simulink model "rpi_driver_blocks"  (R2018b)
settings: Solver=ode45  StartTime=0.0  StopTime=10.0  RelTol=1e-3
PreLoadFcn:
  | Ts = 1e-3
PreSaveFcn:
  | set_param(gcs, 'location', [15 50 815 560])
settings Model: SimulationMode=external  ExtModeTrigDuration=100  Creator=The MathWorks Inc.  LastModifiedBy=benkl
settings DataIOCC: LimitDataPoints=on  SaveFormat=Array
settings OptimizationCC: BlockReduction=off  BooleanDataType=off  LifeSpan=inf
settings DebuggingCC: SaveWithParameterizedLinksMsg=none  UnderspecifiedInitializationDetection=Classic  MergeDetectMultiDrivingBlocksExec=none  SignalResolutionControl=TryResolveAllWithWarning  SFUnexpectedBacktrackingDiag=warning  SFNoUnconditionalDefaultTransitionDiag=warning  SFExecutionAtInitializationDiag=none
settings HardwareCC: ProdBitPerPointer=32  ProdBitPerSizeT=32  ProdBitPerPtrDiffT=32  ProdLargestAtomicFloat=None  ProdIntDivRoundTo=Undefined  ProdEndianess=Unspecified  ProdWordSize=32  ProdHWDeviceType=32-bit Generic  TargetUnknown=on
settings ModelReferenceCC: PropagateSignalLabelsOutOfModel=off
settings SFSimCC: SimUseLocalCustomCode=off
settings RTWCC: RTWUseLocalCustomCode=off
settings CodeAppCC: StateflowObjectComments=on
settings GRTTargetCC: TargetLangStandard=C89/C90 (ANSI)  GeneratePreprocessorConditionals=Disable all
settings ConfigComp: CovMetricSettings=dw  CovHtmlReporting=on  CovSaveCumulativeToWorkspaceVar=on  CovSaveSingleToWorkspaceVar=on  CovExternalEMLEnable=off  CovSFcnEnable=off

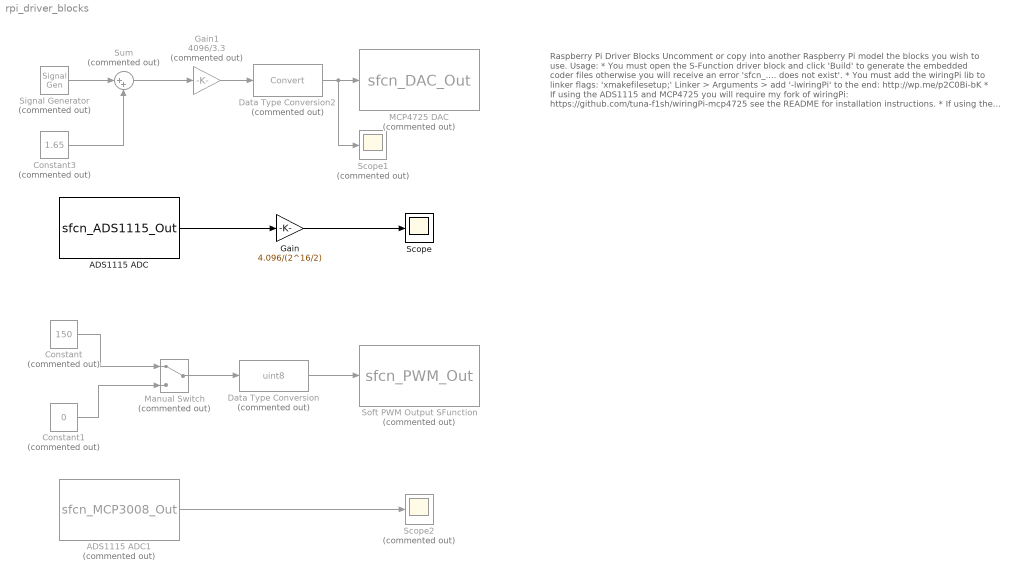
== system rpi_driver_blocks ==
  note: Raspberry Pi Driver Blocks
      |
      | Uncomment or copy into another Raspberry Pi model the blocks you wish to use.
      |
      | Usage:
      |
      | * You must open the S-Function driver block and click 'Build' to generate the embedded coder files
      | otherwise you will receive an error 'sfcn_.... does not exist'.
      |
      | * You must add the wiringPi lib to linker flags: 'xmakefilesetup;' Linker > Arguments > add '-lwiringPi' to the end:
      | http://wp.me/p2C0Bi-bK
      |
      | * If using the ADS1115 and MCP4725 you will require my fork of wiringPi: https://github.com/tuna-f1sh/wiringPi-mcp4725
      | see the README for installation instructions.
      |
      | * If using the PWM block, you will need to enable SPI in Raspbian - see:
      | http://uk.mathworks.com/help/supportpkg/raspberrypiio/examples/analog-input-using-spi.html or enable via SSH
      |
      | * The scopes work in real-time on the Pi to see the correct data is going to/coming from blocks.
      |
      | * The discrete timestep is set to 'Ts' throughout the model. This is initialised as 1e-3s at model load - it seems to be the
      | sweet spot for performance/usage. Remember to consider quantisation that this can create with signals driving the blocks.
      |
      | Notes:
      |
      | * wiringPi softPWM: https://projects.drogon.net/raspberry-pi/wiringpi/software-pwm-library/
      |
      | * Do not sure both ADC blocks at once without changing the wiringPi 'pin' assignment - it won't work.
      |
      | www.jbrengineering.co.uk - @j_whittington - 2015
  ADS1115 ADC : S-Function  InitFcn=try, set_param(gcb,'FunctionName','sfcn_ADS1115_Out'), end  FunctionName=sfcn_ADS1115_Out  Parameters=uint8(0)  SFunctionModules=sfcn_ADS1115_Out_wrapper  SFunctionDeploymentMode=off  EnableBusSupport=off  mask(S-Function Builder){}
      mask init:
      | val = [[.9  0.75 0.75 1 1 .9 .9 1]',[1 1 0.75 0.75 .9 .9 1 .9]'];try , sys = get_param(gcb,'SfunBuilderFcnName');if isempty(sys), sys = get_param(gcb,'FunctionName'); end,catch, sys = get_param(gcb,'FunctionName'); end
      settings: CopyFcn=set_param(gcbh,'LinkStatus','none')  PreSaveFcn=try, set_param(gcb,'FunctionName','sfcn_ADS1115_Out'), end  OpenFcn=sfunctionwizard(gcbh)
      mask Display: plot(val(:,1),val(:,2)),disp(sys), port_label('output',1,'y0')
  ADS1115 ADC1 : S-Function  Commented=on  InitFcn=try, set_param(gcb,'FunctionName','sfcn_MCP3008_Out'), end  FunctionName=sfcn_MCP3008_Out  Parameters=uint8(0)  SFunctionModules=sfcn_MCP3008_Out_wrapper  SFunctionDeploymentMode=off  EnableBusSupport=off  mask(S-Function Builder){}
      mask init: same as rpi_driver_blocks/ADS1115 ADC
      settings: CopyFcn=set_param(gcbh,'LinkStatus','none')  PreSaveFcn=try, set_param(gcb,'FunctionName','sfcn_MCP3008_Out'), end  OpenFcn=sfunctionwizard(gcbh)
      mask Display: plot(val(:,1),val(:,2)),disp(sys), port_label('output',1,'y0')
  Constant : Constant  Commented=on  Value=150
  Constant1 : Constant  Commented=on  Value=0
  Constant3 : Constant  Commented=on  Value=1.65  SampleTime=Ts
  Data Type Conversion : DataTypeConversion  Commented=on  OutDataTypeStr=uint8
  Data Type Conversion2 : DataTypeConversion  Commented=on
  Gain : Gain  Gain=4.096/(2^16/2)  SampleTime=Ts
  Gain1 : Gain  Commented=on  Gain=4096/3.3  SampleTime=Ts
  MCP4725 DAC : S-Function  Commented=on  InitFcn=try, set_param(gcb,'FunctionName','sfcn_DAC_Out'), end  FunctionName=sfcn_DAC_Out  Parameters=uint8(0)  SFunctionModules=sfcn_DAC_Out_wrapper  SFunctionDeploymentMode=off  EnableBusSupport=off  mask(S-Function Builder){}
      mask init: same as rpi_driver_blocks/ADS1115 ADC
      settings: CopyFcn=set_param(gcbh,'LinkStatus','none')  PreSaveFcn=try, set_param(gcb,'FunctionName','sfcn_DAC_Out'), end  OpenFcn=sfunctionwizard(gcbh)
      mask Display: plot(val(:,1),val(:,2)),disp(sys), port_label('input',1,'u0')
  Manual Switch : ManualSwitch  Commented=on
  Scope : Scope
  Scope1 : Scope  Commented=on
  Scope2 : Scope  Commented=on
  Signal Generator : SignalGenerator  Commented=on  Amplitude=1.65  Frequency=5
  Soft PWM Output SFunction : S-Function  Commented=on  InitFcn=try, set_param(gcb,'FunctionName','sfcn_PWM_Out'), end  FunctionName=sfcn_PWM_Out  Parameters=uint8(0)  SFunctionModules=sfcn_PWM_Out_wrapper  SFunctionDeploymentMode=off  EnableBusSupport=off  mask(S-Function Builder){}
      mask init: same as rpi_driver_blocks/ADS1115 ADC
      settings: CopyFcn=set_param(gcbh,'LinkStatus','none')  PreSaveFcn=try, set_param(gcb,'FunctionName','sfcn_PWM_Out'), end  OpenFcn=sfunctionwizard(gcbh)
      mask Display: plot(val(:,1),val(:,2)),disp(sys), port_label('input',1,'in')
  Sum : Sum  Commented=on  Inputs=|++
  wires:
  Constant/1 -> Manual Switch/1
  Constant1/1 -> Manual Switch/2
  Manual Switch/1 -> Data Type Conversion/1
  Data Type Conversion/1 -> Soft PWM Output SFunction/1
  Gain/1 -> Scope/1
  ADS1115 ADC/1 -> Gain/1
  Data Type Conversion2/1 -> MCP4725 DAC/1, Scope1/1
  Sum/1 -> Gain1/1
  Signal Generator/1 -> Sum/1
  Constant3/1 -> Sum/2
  Gain1/1 -> Data Type Conversion2/1
  ADS1115 ADC1/1 -> Scope2/1
